simulink model "MCU_FOC"  (R2022b)
settings: Solver=FixedStepDiscrete  StartTime=0.0  StopTime=10.0  FixedStep=0.0001  RelTol=1e-3
values from neighbouring files (symbols this model uses):
  C_FOC_DecoupleEn_u8 = 0.0    [MCU_FOC_Sldd.sldd]    (also in MCU_FOC_Sldd_objects.m = myPackage.Parameter)
  C_FOC_DecoupleUdCoeff_f32 = 0.0    [MCU_FOC_Sldd.sldd]    (also in MCU_FOC_Sldd_objects.m = myPackage.Parameter)
  C_FOC_DecoupleUeCoeff_f32 = 0.0    [MCU_FOC_Sldd.sldd]    (also in MCU_FOC_Sldd_objects.m = myPackage.Parameter)
  C_FOC_DecoupleUqCoeff_f32 = 0.0    [MCU_FOC_Sldd.sldd]    (also in MCU_FOC_Sldd_objects.m = myPackage.Parameter)
  C_FOC_DPWMEN_u8 = 0.0    [MCU_FOC_Sldd.sldd]    (also in MCU_FOC_Sldd_objects.m = myPackage.Parameter)
  C_FOC_IgnoreShunt_u8 = 0.0    [MCU_FOC_Sldd.sldd]    (also in MCU_FOC_Sldd_objects.m = myPackage.Parameter)
  C_FOC_ThetaOffsetCoeff_f32 = 0.0    [MCU_FOC_Sldd.sldd]    (also in MCU_FOC_Sldd_objects.m = myPackage.Parameter)
undefined symbols (not defined in the file or in its folder): ABC_SAMPLE, ANALOG, cAgeingMode, cParaRecogMode, cSingleBoardMode, cVvvfOpenMode, MAIN_CPU_FRE, ParamCfg_BaseSpeed_u16, ParamCfg_CommandSource_u16, ParamCfg_IdKi_u16, ParamCfg_IdKp_u16, ParamCfg_IdStep1_u16, ParamCfg_IdStep2_u16, ParamCfg_IqKi_u16, ParamCfg_IqKp_u16, ParamCfg_IqStep_u16, ParamCfg_MotorLsd_u16, ParamCfg_MotorNp_u16, ParamCfg_MotorUlsq_u16, ParamCfg_PwmFreqHigh_u16, ParamCfg_PwmFreqLow_u16, ParamCfg_Pwmprdchgen_u16, ParamCfg_RotateNp_u16, ParamCfg_RotorFlux_u16, ParamCfg_SampleMode_u16, TESTBED
libraries: simulink x40, YS_UserDefined_Library x17
(part 1 of 2)
settings Model: DataDictionary=MCU_FOC_Sldd.sldd  Creator=ZYH  LastModifiedBy=ZYH
settings OptimizationCC: DefaultParameterBehavior=Inlined  EnhancedBackFolding=on  PassReuseOutputArgsAs=Individual arguments  ZeroExternalMemoryAtStartup=off  ZeroInternalMemoryAtStartup=off  OptimizeBlockOrder=speed  DifferentSizesBufferReuse=on  OptimizationCustomize=off  EfficientTunableParamExpr=on
settings DebuggingCC: ParameterTunabilityLossMsg=error
settings SFSimCC: MATLABDynamicMemAlloc=off
settings RTWCC: Description=Embedded Coder  SystemTargetFile=ert.tlc  GenCodeOnly=on  TemplateMakefile=ert_default_tmf
settings CodeAppCC: ForceParamTrailComments=on  IgnoreCustomStorageClasses=off  OperatorAnnotations=on  SimulinkDataObjDesc=on  SFDataObjDesc=on  InsertBlockDesc=on
settings ERTTargetCC: TargetLangStandard=C99 (ISO)  GenerateSampleERTMain=on  InlinedParameterPlacement=NonHierarchical  ERTCustomFileTemplate=example_file_process.tlc

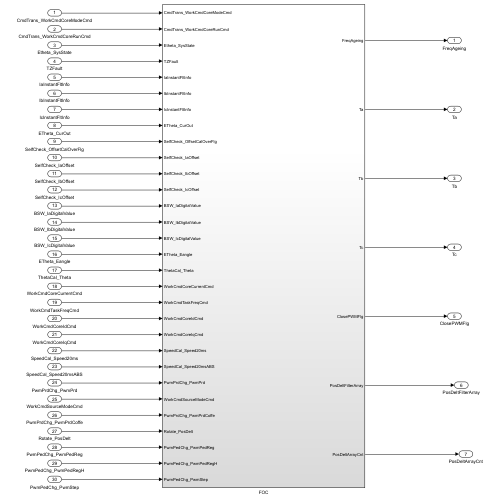
[thumbnail: Simulink's stored preview of the top-level diagram]
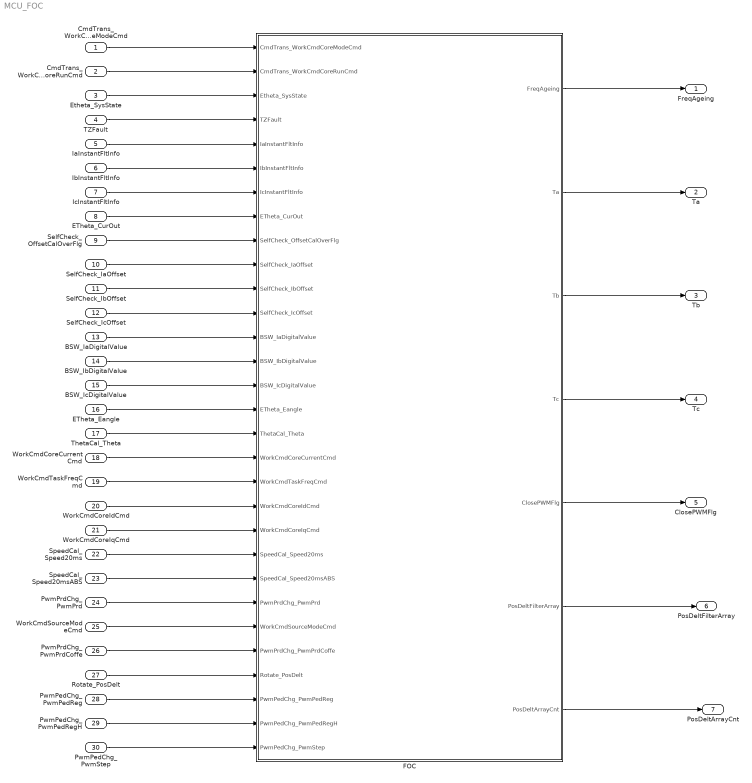
== system MCU_FOC ==
  CmdTrans_WorkCmdCoreModeCmd : Inport
  CmdTrans_WorkCmdCoreRunCmd : Inport  Port=2
  Etheta_SysState : Inport  Port=3
  TZFault : Inport  Port=4
  IaInstantFltInfo : Inport  Port=5
  IbInstantFltInfo : Inport  Port=6
  IcInstantFltInfo : Inport  Port=7
  ETheta_CurOut : Inport  Port=8
  SelfCheck_OffsetCalOverFlg : Inport  Port=9
  SelfCheck_IaOffset : Inport  Port=10
  SelfCheck_IbOffset : Inport  Port=11
  SelfCheck_IcOffset : Inport  Port=12
  BSW_IaDigitalValue : Inport  Port=13
  BSW_IbDigitalValue : Inport  Port=14
  BSW_IcDigitalValue : Inport  Port=15
  ETheta_Eangle : Inport  Port=16
  ThetaCal_Theta : Inport  Port=17
  WorkCmdCoreCurrentCmd : Inport  Port=18
  WorkCmdTaskFreqCmd : Inport  Port=19
  WorkCmdCoreIdCmd : Inport  Port=20
  WorkCmdCoreIqCmd : Inport  Port=21
  SpeedCal_Speed20ms : Inport  Port=22
  SpeedCal_Speed20msABS : Inport  Port=23
  PwmPrdChg_PwmPrd : Inport  Port=24
  WorkCmdSourceModeCmd : Inport  Port=25
  PwmPrdChg_PwmPrdCoffe : Inport  Port=26
  Rotate_PosDelt : Inport  Port=27
  PwmPedChg_PwmPedReg : Inport  Port=28
  PwmPedChg_PwmPedRegH : Inport  Port=29
  PwmPedChg_PwmStep : Inport  Port=30
  FOC : Subsystem
  FreqAgeing : Outport
  Ta : Outport  Port=2
  Tb : Outport  Port=3
  Tc : Outport  Port=4
  ClosePWMFlg : Outport  Port=5
  PosDeltFilterArray : Outport  Port=6
  PosDeltArrayCnt : Outport  Port=7
  wires:
  FOC/2(Ta) -> Ta/1
  WorkCmdCoreIqCmd/1 -> FOC/21(WorkCmdCoreIqCmd)
  WorkCmdCoreCurrentCmd/1 -> FOC/18(WorkCmdCoreCurrentCmd)
  FOC/1(FreqAgeing) -> FreqAgeing/1
  WorkCmdTaskFreqCmd/1 -> FOC/19(WorkCmdTaskFreqCmd)
  SelfCheck_IaOffset/1 -> FOC/10(SelfCheck_IaOffset)
  WorkCmdCoreIdCmd/1 -> FOC/20(WorkCmdCoreIdCmd)
  SelfCheck_IbOffset/1 -> FOC/11(SelfCheck_IbOffset)
  IcInstantFltInfo/1 -> FOC/7(IcInstantFltInfo)
  ETheta_Eangle/1 -> FOC/16(ETheta_Eangle)
  SelfCheck_OffsetCalOverFlg/1 -> FOC/9(SelfCheck_OffsetCalOverFlg)
  ThetaCal_Theta/1 -> FOC/17(ThetaCal_Theta)
  TZFault/1 -> FOC/4(TZFault)
  PwmPedChg_PwmPedReg/1 -> FOC/28(PwmPedChg_PwmPedReg)
  PwmPrdChg_PwmPrd/1 -> FOC/24(PwmPrdChg_PwmPrd)
  Rotate_PosDelt/1 -> FOC/27(Rotate_PosDelt)
  SpeedCal_Speed20ms/1 -> FOC/22(SpeedCal_Speed20ms)
  FOC/4(Tc) -> Tc/1
  BSW_IaDigitalValue/1 -> FOC/13(BSW_IaDigitalValue)
  BSW_IbDigitalValue/1 -> FOC/14(BSW_IbDigitalValue)
  PwmPedChg_PwmPedRegH/1 -> FOC/29(PwmPedChg_PwmPedRegH)
  PwmPrdChg_PwmPrdCoffe/1 -> FOC/26(PwmPrdChg_PwmPrdCoffe)
  WorkCmdSourceModeCmd/1 -> FOC/25(WorkCmdSourceModeCmd)
  ETheta_CurOut/1 -> FOC/8(ETheta_CurOut)
  SpeedCal_Speed20msABS/1 -> FOC/23(SpeedCal_Speed20msABS)
  BSW_IcDigitalValue/1 -> FOC/15(BSW_IcDigitalValue)
  Etheta_SysState/1 -> FOC/3(Etheta_SysState)
  SelfCheck_IcOffset/1 -> FOC/12(SelfCheck_IcOffset)
  IaInstantFltInfo/1 -> FOC/5(IaInstantFltInfo)
  CmdTrans_WorkCmdCoreRunCmd/1 -> FOC/2(CmdTrans_WorkCmdCoreRunCmd)
  IbInstantFltInfo/1 -> FOC/6(IbInstantFltInfo)
  CmdTrans_WorkCmdCoreModeCmd/1 -> FOC/1(CmdTrans_WorkCmdCoreModeCmd)
  FOC/3(Tb) -> Tb/1
  FOC/5(ClosePWMFlg) -> ClosePWMFlg/1
  PwmPedChg_PwmStep/1 -> FOC/30(PwmPedChg_PwmStep)
  FOC/6(PosDeltFilterArray) -> PosDeltFilterArray/1
  FOC/7(PosDeltArrayCnt) -> PosDeltArrayCnt/1

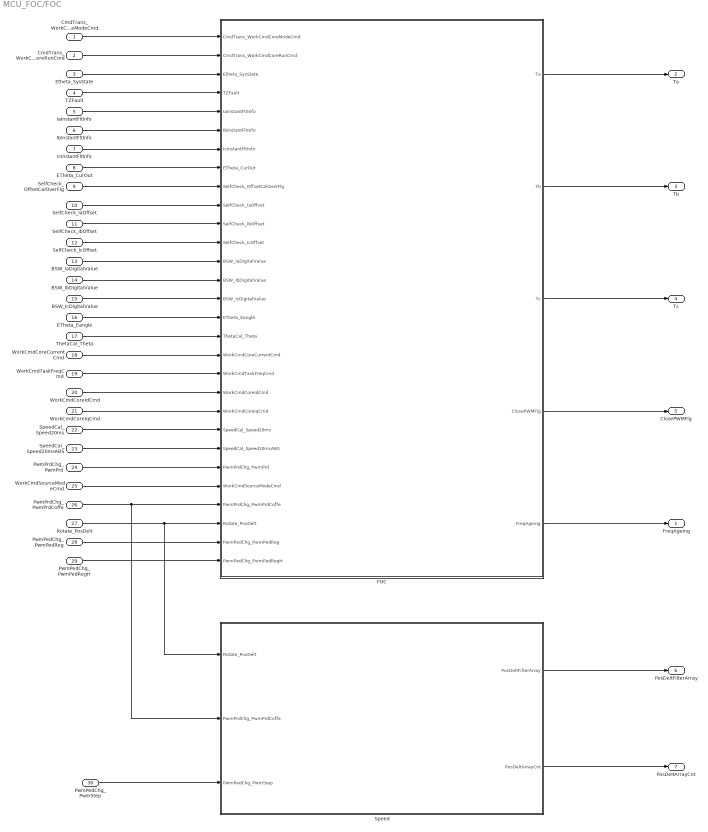
== system MCU_FOC/FOC ==
  CmdTrans_WorkCmdCoreModeCmd : Inport
  CmdTrans_WorkCmdCoreRunCmd : Inport  Port=2
  Etheta_SysState : Inport  Port=3
  TZFault : Inport  Port=4
  IaInstantFltInfo : Inport  Port=5
  IbInstantFltInfo : Inport  Port=6
  IcInstantFltInfo : Inport  Port=7
  ETheta_CurOut : Inport  Port=8
  SelfCheck_OffsetCalOverFlg : Inport  Port=9
  SelfCheck_IaOffset : Inport  Port=10
  SelfCheck_IbOffset : Inport  Port=11
  SelfCheck_IcOffset : Inport  Port=12
  BSW_IaDigitalValue : Inport  Port=13
  BSW_IbDigitalValue : Inport  Port=14
  BSW_IcDigitalValue : Inport  Port=15
  ETheta_Eangle : Inport  Port=16
  ThetaCal_Theta : Inport  Port=17
  WorkCmdCoreCurrentCmd : Inport  Port=18
  WorkCmdTaskFreqCmd : Inport  Port=19
  WorkCmdCoreIdCmd : Inport  Port=20
  WorkCmdCoreIqCmd : Inport  Port=21
  SpeedCal_Speed20ms : Inport  Port=22
  SpeedCal_Speed20msABS : Inport  Port=23
  PwmPrdChg_PwmPrd : Inport  Port=24
  WorkCmdSourceModeCmd : Inport  Port=25
  PwmPrdChg_PwmPrdCoffe : Inport  Port=26
  Rotate_PosDelt : Inport  Port=27
  PwmPedChg_PwmPedReg : Inport  Port=28
  PwmPedChg_PwmPedRegH : Inport  Port=29
  PwmPedChg_PwmStep : Inport  Port=30
  FOC : Subsystem
  Speed : Subsystem
  FreqAgeing : Outport
  Ta : Outport  Port=2
  Tb : Outport  Port=3
  Tc : Outport  Port=4
  ClosePWMFlg : Outport  Port=5
  PosDeltFilterArray : Outport  Port=6
  PosDeltArrayCnt : Outport  Port=7
  wires:
  CmdTrans_WorkCmdCoreModeCmd/1 -> FOC/1(CmdTrans_WorkCmdCoreModeCmd)
  CmdTrans_WorkCmdCoreRunCmd/1 -> FOC/2(CmdTrans_WorkCmdCoreRunCmd)
  Etheta_SysState/1 -> FOC/3(Etheta_SysState)
  TZFault/1 -> FOC/4(TZFault)
  IaInstantFltInfo/1 -> FOC/5(IaInstantFltInfo)
  IbInstantFltInfo/1 -> FOC/6(IbInstantFltInfo)
  IcInstantFltInfo/1 -> FOC/7(IcInstantFltInfo)
  ETheta_CurOut/1 -> FOC/8(ETheta_CurOut)
  SelfCheck_OffsetCalOverFlg/1 -> FOC/9(SelfCheck_OffsetCalOverFlg)
  SelfCheck_IaOffset/1 -> FOC/10(SelfCheck_IaOffset)
  SelfCheck_IbOffset/1 -> FOC/11(SelfCheck_IbOffset)
  SelfCheck_IcOffset/1 -> FOC/12(SelfCheck_IcOffset)
  BSW_IaDigitalValue/1 -> FOC/13(BSW_IaDigitalValue)
  BSW_IbDigitalValue/1 -> FOC/14(BSW_IbDigitalValue)
  BSW_IcDigitalValue/1 -> FOC/15(BSW_IcDigitalValue)
  ETheta_Eangle/1 -> FOC/16(ETheta_Eangle)
  ThetaCal_Theta/1 -> FOC/17(ThetaCal_Theta)
  WorkCmdCoreCurrentCmd/1 -> FOC/18(WorkCmdCoreCurrentCmd)
  WorkCmdTaskFreqCmd/1 -> FOC/19(WorkCmdTaskFreqCmd)
  WorkCmdCoreIdCmd/1 -> FOC/20(WorkCmdCoreIdCmd)
  WorkCmdCoreIqCmd/1 -> FOC/21(WorkCmdCoreIqCmd)
  SpeedCal_Speed20ms/1 -> FOC/22(SpeedCal_Speed20ms)
  SpeedCal_Speed20msABS/1 -> FOC/23(SpeedCal_Speed20msABS)
  PwmPrdChg_PwmPrd/1 -> FOC/24(PwmPrdChg_PwmPrd)
  WorkCmdSourceModeCmd/1 -> FOC/25(WorkCmdSourceModeCmd)
  PwmPrdChg_PwmPrdCoffe/1 -> Speed/2(PwmPrdChg_PwmPrdCoffe), FOC/26(PwmPrdChg_PwmPrdCoffe)
  Rotate_PosDelt/1 -> Speed/1(Rotate_PosDelt), FOC/27(Rotate_PosDelt)
  PwmPedChg_PwmPedReg/1 -> FOC/28(PwmPedChg_PwmPedReg)
  PwmPedChg_PwmPedRegH/1 -> FOC/29(PwmPedChg_PwmPedRegH)
  FOC/1(Ta) -> Ta/1
  FOC/2(Tb) -> Tb/1
  FOC/3(Tc) -> Tc/1
  FOC/4(ClosePWMFlg) -> ClosePWMFlg/1
  FOC/5(FreqAgeing) -> FreqAgeing/1
  PwmPedChg_PwmStep/1 -> Speed/3(PwmPedChg_PwmStep)
  Speed/1(PosDeltFilterArray) -> PosDeltFilterArray/1
  Speed/2(PosDeltArrayCnt) -> PosDeltArrayCnt/1

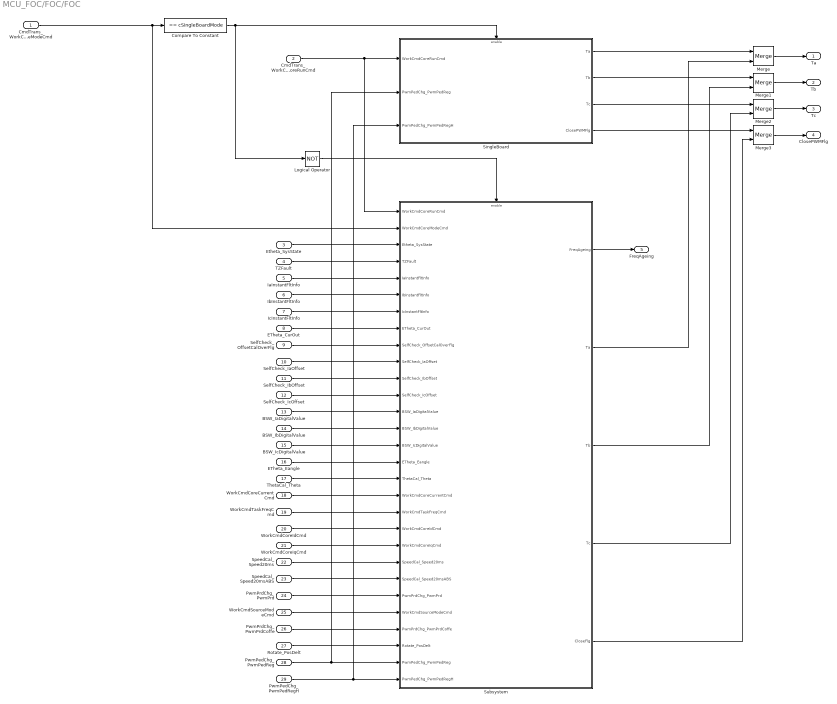
== system MCU_FOC/FOC/FOC ==
  CmdTrans_WorkCmdCoreModeCmd : Inport
  CmdTrans_WorkCmdCoreRunCmd : Inport  Port=2
  Etheta_SysState : Inport  Port=3
  TZFault : Inport  Port=4
  IaInstantFltInfo : Inport  Port=5
  IbInstantFltInfo : Inport  Port=6
  IcInstantFltInfo : Inport  Port=7
  ETheta_CurOut : Inport  Port=8
  SelfCheck_OffsetCalOverFlg : Inport  Port=9
  SelfCheck_IaOffset : Inport  Port=10
  SelfCheck_IbOffset : Inport  Port=11
  SelfCheck_IcOffset : Inport  Port=12
  BSW_IaDigitalValue : Inport  Port=13
  BSW_IbDigitalValue : Inport  Port=14
  BSW_IcDigitalValue : Inport  Port=15
  ETheta_Eangle : Inport  Port=16
  ThetaCal_Theta : Inport  Port=17
  WorkCmdCoreCurrentCmd : Inport  Port=18
  WorkCmdTaskFreqCmd : Inport  Port=19
  WorkCmdCoreIdCmd : Inport  Port=20
  WorkCmdCoreIqCmd : Inport  Port=21
  SpeedCal_Speed20ms : Inport  Port=22
  SpeedCal_Speed20msABS : Inport  Port=23
  PwmPrdChg_PwmPrd : Inport  Port=24
  WorkCmdSourceModeCmd : Inport  Port=25
  PwmPrdChg_PwmPrdCoffe : Inport  Port=26
  Rotate_PosDelt : Inport  Port=27
  PwmPedChg_PwmPedReg : Inport  Port=28
  PwmPedChg_PwmPedRegH : Inport  Port=29
  Compare To Constant : simulink/Logic and Bit Operations/Compare To Constant  relop===  const=cSingleBoardMode  OutDataTypeStr=boolean
  Logical Operator : Logic  Operator=NOT  AllPortsSameDT=off  OutDataTypeStr=boolean
  Merge{,1..3} (4 alike) : Merge
  SingleBoard : Subsystem  TreatAsAtomicUnit=on
  Subsystem : Subsystem
  Ta : Outport
  Tb : Outport  Port=2
  Tc : Outport  Port=3
  ClosePWMFlg : Outport  Port=4
  FreqAgeing : Outport  Port=5
  wires:
  SpeedCal_Speed20ms/1 -> Subsystem/22(SpeedCal_Speed20ms)
  Etheta_SysState/1 -> Subsystem/3(Etheta_SysState)
  WorkCmdCoreIdCmd/1 -> Subsystem/20(WorkCmdCoreIdCmd)
  SelfCheck_OffsetCalOverFlg/1 -> Subsystem/9(SelfCheck_OffsetCalOverFlg)
  SelfCheck_IbOffset/1 -> Subsystem/11(SelfCheck_IbOffset)
  PwmPrdChg_PwmPrdCoffe/1 -> Subsystem/26(PwmPrdChg_PwmPrdCoffe)
  Compare To Constant/1 -> SingleBoard/Enable, Logical Operator/1
  ETheta_Eangle/1 -> Subsystem/16(ETheta_Eangle)
  CmdTrans_WorkCmdCoreModeCmd/1 -> Compare To Constant/1, Subsystem/2(WorkCmdCoreModeCmd)
  SingleBoard/3(Tc) -> Merge2/1
  PwmPedChg_PwmPedRegH/1 -> SingleBoard/3(PwmPedChg_PwmPedRegH), Subsystem/29(PwmPedChg_PwmPedRegH)
  ETheta_CurOut/1 -> Subsystem/8(ETheta_CurOut)
  CmdTrans_WorkCmdCoreRunCmd/1 -> Subsystem/1(WorkCmdCoreRunCmd), SingleBoard/1(WorkCmdCoreRunCmd)
  SelfCheck_IcOffset/1 -> Subsystem/12(SelfCheck_IcOffset)
  WorkCmdTaskFreqCmd/1 -> Subsystem/19(WorkCmdTaskFreqCmd)
  PwmPedChg_PwmPedReg/1 -> SingleBoard/2(PwmPedChg_PwmPedReg), Subsystem/28(PwmPedChg_PwmPedReg)
  SingleBoard/1(Ta) -> Merge/1
  PwmPrdChg_PwmPrd/1 -> Subsystem/24(PwmPrdChg_PwmPrd)
  BSW_IaDigitalValue/1 -> Subsystem/13(BSW_IaDigitalValue)
  BSW_IcDigitalValue/1 -> Subsystem/15(BSW_IcDigitalValue)
  ThetaCal_Theta/1 -> Subsystem/17(ThetaCal_Theta)
  IbInstantFltInfo/1 -> Subsystem/6(IbInstantFltInfo)
  IaInstantFltInfo/1 -> Subsystem/5(IaInstantFltInfo)
  Merge/1 -> Ta/1
  Subsystem/3(Tb) -> Merge1/2
  WorkCmdCoreIqCmd/1 -> Subsystem/21(WorkCmdCoreIqCmd)
  SelfCheck_IaOffset/1 -> Subsystem/10(SelfCheck_IaOffset)
  IcInstantFltInfo/1 -> Subsystem/7(IcInstantFltInfo)
  Logical Operator/1 -> Subsystem/Enable
  WorkCmdCoreCurrentCmd/1 -> Subsystem/18(WorkCmdCoreCurrentCmd)
  Rotate_PosDelt/1 -> Subsystem/27(Rotate_PosDelt)
  TZFault/1 -> Subsystem/4(TZFault)
  SpeedCal_Speed20msABS/1 -> Subsystem/23(SpeedCal_Speed20msABS)
  BSW_IbDigitalValue/1 -> Subsystem/14(BSW_IbDigitalValue)
  Subsystem/4(Tc) -> Merge2/2
  Subsystem/1(FreqAgeing) -> FreqAgeing/1
  SingleBoard/4(ClosePWMFlg) -> Merge3/1
  Subsystem/2(Ta) -> Merge/2
  SingleBoard/2(Tb) -> Merge1/1
  Subsystem/5(CloseFlg) -> Merge3/2
  WorkCmdSourceModeCmd/1 -> Subsystem/25(WorkCmdSourceModeCmd)
  Merge1/1 -> Tb/1
  Merge2/1 -> Tc/1
  Merge3/1 -> ClosePWMFlg/1

== system MCU_FOC/FOC/Speed ==
  Rotate_PosDelt : Inport
  PwmPrdChg_PwmPrdCoffe : Inport  Port=2
  PwmPedChg_PwmStep : Inport  Port=3
  Chart : Stateflow chart  TreatAsAtomicUnit=on
  Data Type Conversion : DataTypeConversion  OutDataTypeStr=uint8  SaturateOnIntegerOverflow=off  RndMeth=Floor
  PosDeltFilterArray : Outport
  PosDeltArrayCnt : Outport  Port=2
  wires:
  PwmPedChg_PwmStep/1 -> Data Type Conversion/1
  Data Type Conversion/1 -> Chart/1(PWMStep)
  PwmPrdChg_PwmPrdCoffe/1 -> Chart/2(PwmPrdchgCoffe)
  Chart/1(PosDeltFilterArray) -> PosDeltFilterArray/1
  Chart/2(PosDeltArrayCnt) -> PosDeltArrayCnt/1
  Rotate_PosDelt/1 -> Chart/3(PosDelt)

== system MCU_FOC/FOC/FOC/SingleBoard ==
  WorkCmdCoreRunCmd : Inport
  PwmPedChg_PwmPedReg : Inport  Port=2
  PwmPedChg_PwmPedRegH : Inport  Port=3
  Enable : EnablePort
  ClosePWM : Subsystem  TreatAsAtomicUnit=on
  Compare To Constant : simulink/Logic and Bit Operations/Compare To Constant  relop===  const=true  OutDataTypeStr=boolean
  Compare To Constant1 : simulink/Logic and Bit Operations/Compare To Constant  relop===  const=false  OutDataTypeStr=boolean
  ForcePWM : Subsystem  TreatAsAtomicUnit=on
  Ta : Outport
  Tb : Outport  Port=2
  Tc : Outport  Port=3
  ClosePWMFlg : Outport  Port=4
  wires:
  WorkCmdCoreRunCmd/1 -> Compare To Constant1/1, Compare To Constant/1
  Compare To Constant/1 -> ForcePWM/Enable
  Compare To Constant1/1 -> ClosePWM/Enable
  PwmPedChg_PwmPedRegH/1 -> ForcePWM/2(PwmPedChg_PwmPedRegH)
  PwmPedChg_PwmPedReg/1 -> ForcePWM/1(PwmPedChg_PwmPedReg)
  ForcePWM/1(Ta) -> Ta/1
  ForcePWM/2(Tb) -> Tb/1
  ForcePWM/3(Tc) -> Tc/1
  ClosePWM/1(ClosePWMFlg) -> ClosePWMFlg/1

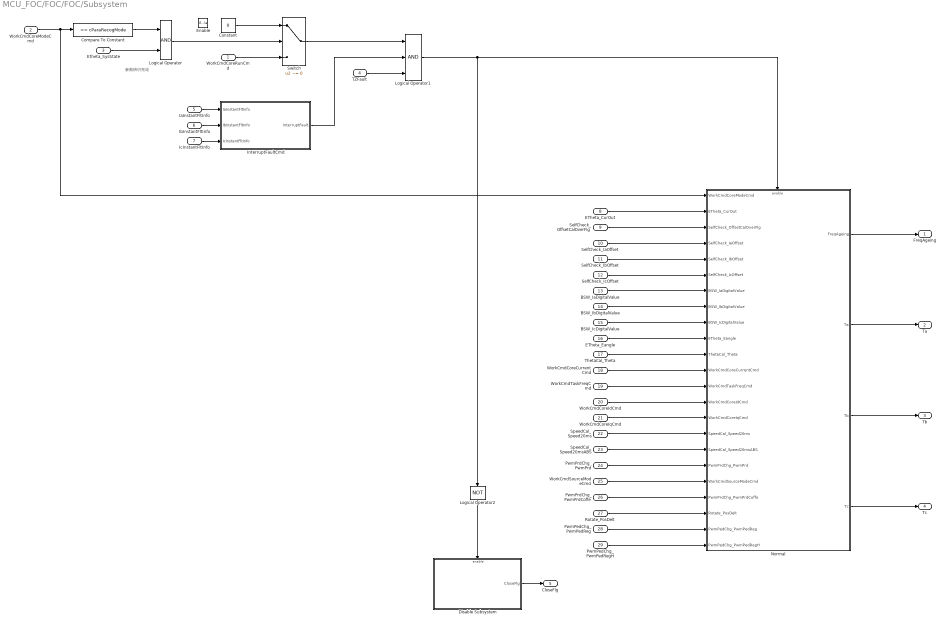
== system MCU_FOC/FOC/FOC/Subsystem ==
  note: 参数辨识完成
  WorkCmdCoreRunCmd : Inport
  WorkCmdCoreModeCmd : Inport  Port=2
  Etheta_SysState : Inport  Port=3
  TZFault : Inport  Port=4
  IaInstantFltInfo : Inport  Port=5
  IbInstantFltInfo : Inport  Port=6
  IcInstantFltInfo : Inport  Port=7
  ETheta_CurOut : Inport  Port=8
  SelfCheck_OffsetCalOverFlg : Inport  Port=9
  SelfCheck_IaOffset : Inport  Port=10
  SelfCheck_IbOffset : Inport  Port=11
  SelfCheck_IcOffset : Inport  Port=12
  BSW_IaDigitalValue : Inport  Port=13
  BSW_IbDigitalValue : Inport  Port=14
  BSW_IcDigitalValue : Inport  Port=15
  ETheta_Eangle : Inport  Port=16
  ThetaCal_Theta : Inport  Port=17
  WorkCmdCoreCurrentCmd : Inport  Port=18
  WorkCmdTaskFreqCmd : Inport  Port=19
  WorkCmdCoreIdCmd : Inport  Port=20
  WorkCmdCoreIqCmd : Inport  Port=21
  SpeedCal_Speed20ms : Inport  Port=22
  SpeedCal_Speed20msABS : Inport  Port=23
  PwmPrdChg_PwmPrd : Inport  Port=24
  WorkCmdSourceModeCmd : Inport  Port=25
  PwmPrdChg_PwmPrdCoffe : Inport  Port=26
  Rotate_PosDelt : Inport  Port=27
  PwmPedChg_PwmPedReg : Inport  Port=28
  PwmPedChg_PwmPedRegH : Inport  Port=29
  Enable : EnablePort
  Compare To Constant : simulink/Logic and Bit Operations/Compare To Constant  relop===  const=cParaRecogMode  OutDataTypeStr=boolean
  Constant : Constant  Value=0  OutDataTypeStr=uint8
  Disable Subsystem : Subsystem  TreatAsAtomicUnit=on
  InterruptFaultCmd : Subsystem
  Logical Operator : Logic  AllPortsSameDT=off  OutDataTypeStr=boolean
  Logical Operator1 : Logic  Inputs=3  AllPortsSameDT=off  OutDataTypeStr=boolean
  Logical Operator2 : Logic  Operator=NOT  Inputs=3  AllPortsSameDT=off  OutDataTypeStr=boolean
  Normal : Subsystem
  Switch : Switch  Criteria=u2 ~= 0  SaturateOnIntegerOverflow=off  InputSameDT=off
  FreqAgeing : Outport
  Ta : Outport  Port=2
  Tb : Outport  Port=3
  Tc : Outport  Port=4
  CloseFlg : Outport  Port=5
  wires:
  Compare To Constant/1 -> Logical Operator/1
  Etheta_SysState/1 -> Logical Operator/2
  Logical Operator/1 -> Switch/2
  Constant/1 -> Switch/1
  WorkCmdCoreRunCmd/1 -> Switch/3
  Switch/1 -> Logical Operator1/1
  InterruptFaultCmd/1(InterruptFault) -> Logical Operator1/2
  TZFault/1 -> Logical Operator1/3
  Logical Operator1/1 -> Logical Operator2/1, Normal/Enable
  Logical Operator2/1 -> Disable Subsystem/Enable
  IaInstantFltInfo/1 -> InterruptFaultCmd/1(IaInstantFltInfo)
  IbInstantFltInfo/1 -> InterruptFaultCmd/2(IbInstantFltInfo)
  IcInstantFltInfo/1 -> InterruptFaultCmd/3(IcInstantFltInfo)
  ETheta_CurOut/1 -> Normal/2(ETheta_CurOut)
  SelfCheck_IbOffset/1 -> Normal/5(SelfCheck_IbOffset)
  SelfCheck_IaOffset/1 -> Normal/4(SelfCheck_IaOffset)
  SelfCheck_IcOffset/1 -> Normal/6(SelfCheck_IcOffset)
  BSW_IaDigitalValue/1 -> Normal/7(BSW_IaDigitalValue)
  SelfCheck_OffsetCalOverFlg/1 -> Normal/3(SelfCheck_OffsetCalOverFlg)
  BSW_IbDigitalValue/1 -> Normal/8(BSW_IbDigitalValue)
  BSW_IcDigitalValue/1 -> Normal/9(BSW_IcDigitalValue)
  WorkCmdCoreModeCmd/1 -> Normal/1(WorkCmdCoreModeCmd), Compare To Constant/1
  ETheta_Eangle/1 -> Normal/10(ETheta_Eangle)
  ThetaCal_Theta/1 -> Normal/11(ThetaCal_Theta)
  WorkCmdCoreCurrentCmd/1 -> Normal/12(WorkCmdCoreCurrentCmd)
  WorkCmdTaskFreqCmd/1 -> Normal/13(WorkCmdTaskFreqCmd)
  WorkCmdCoreIdCmd/1 -> Normal/14(WorkCmdCoreIdCmd)
  WorkCmdCoreIqCmd/1 -> Normal/15(WorkCmdCoreIqCmd)
  WorkCmdSourceModeCmd/1 -> Normal/19(WorkCmdSourceModeCmd)
  PwmPrdChg_PwmPrdCoffe/1 -> Normal/20(PwmPrdChg_PwmPrdCoffe)
  PwmPrdChg_PwmPrd/1 -> Normal/18(PwmPrdChg_PwmPrd)
  SpeedCal_Speed20msABS/1 -> Normal/17(SpeedCal_Speed20msABS)
  SpeedCal_Speed20ms/1 -> Normal/16(SpeedCal_Speed20ms)
  Rotate_PosDelt/1 -> Normal/21(Rotate_PosDelt)
  Normal/1(FreqAgeing) -> FreqAgeing/1
  PwmPedChg_PwmPedReg/1 -> Normal/22(PwmPedChg_PwmPedReg)
  PwmPedChg_PwmPedRegH/1 -> Normal/23(PwmPedChg_PwmPedRegH)
  Normal/2(Ta) -> Ta/1
  Normal/3(Tb) -> Tb/1
  Normal/4(Tc) -> Tc/1
  Disable Subsystem/1(CloseFlg) -> CloseFlg/1

== system MCU_FOC/FOC/FOC/SingleBoard/ClosePWM ==
  Enable : EnablePort
  Constant : Constant  OutDataTypeStr=uint8
  ClosePWMFlg : Outport
  wires:
  Constant/1 -> ClosePWMFlg/1

== system MCU_FOC/FOC/FOC/SingleBoard/ForcePWM ==
  PwmPedChg_PwmPedReg : Inport
  PwmPedChg_PwmPedRegH : Inport  Port=2
  Enable : EnablePort
  CmapA : Constant  Value=1000  OutDataTypeStr=single
  CmapB : Constant  Value=5000  OutDataTypeStr=single
  CmapC : Constant  Value=1000  OutDataTypeStr=single
  Divide : Product  Inputs=*/
  Divide1 : Product  Inputs=*/
  Divide2 : Product  Inputs=*/
  SVPWMCtrl : Subsystem
  Subsystem : Subsystem
  Ta : Outport
  Tb : Outport  Port=2
  Tc : Outport  Port=3
  wires:
  Divide/1 -> SVPWMCtrl/1(CmapA)
  Divide1/1 -> SVPWMCtrl/2(CmapB)
  Divide2/1 -> SVPWMCtrl/3(CmapC)
  CmapB/1 -> Divide1/1
  CmapC/1 -> Divide2/1
  CmapA/1 -> Divide/1
  Subsystem/1(PwmPrdReg) -> Divide2/2, Divide1/2, Divide/2
  PwmPedChg_PwmPedReg/1 -> SVPWMCtrl/4(PwmPedChg_PwmPedReg)
  PwmPedChg_PwmPedRegH/1 -> SVPWMCtrl/5(PwmPedChg_PwmPedRegH)
  SVPWMCtrl/1(Ta) -> Ta/1
  SVPWMCtrl/2(Tb) -> Tb/1
  SVPWMCtrl/3(Tc) -> Tc/1

== system MCU_FOC/FOC/FOC/Subsystem/Disable Subsystem ==
  Enable : EnablePort
  Constant : Constant  OutDataTypeStr=uint8
  CloseFlg : Outport
  wires:
  Constant/1 -> CloseFlg/1

== system MCU_FOC/FOC/FOC/Subsystem/InterruptFaultCmd ==
  IaInstantFltInfo : Inport
  IbInstantFltInfo : Inport  Port=2
  IcInstantFltInfo : Inport  Port=3
  Compare To Zero : simulink/Logic and Bit Operations/Compare To Zero  relop===  OutDataTypeStr=boolean
  Compare To Zero1 : simulink/Logic and Bit Operations/Compare To Zero  relop===  OutDataTypeStr=boolean
  Compare To Zero2 : simulink/Logic and Bit Operations/Compare To Zero  relop===  OutDataTypeStr=boolean
  Logical Operator : Logic  Inputs=3  AllPortsSameDT=off  OutDataTypeStr=boolean
  InterruptFault : Outport
  wires:
  IaInstantFltInfo/1 -> Compare To Zero/1
  IbInstantFltInfo/1 -> Compare To Zero1/1
  IcInstantFltInfo/1 -> Compare To Zero2/1
  Compare To Zero/1 -> Logical Operator/1
  Compare To Zero1/1 -> Logical Operator/2
  Compare To Zero2/1 -> Logical Operator/3
  Logical Operator/1 -> InterruptFault/1

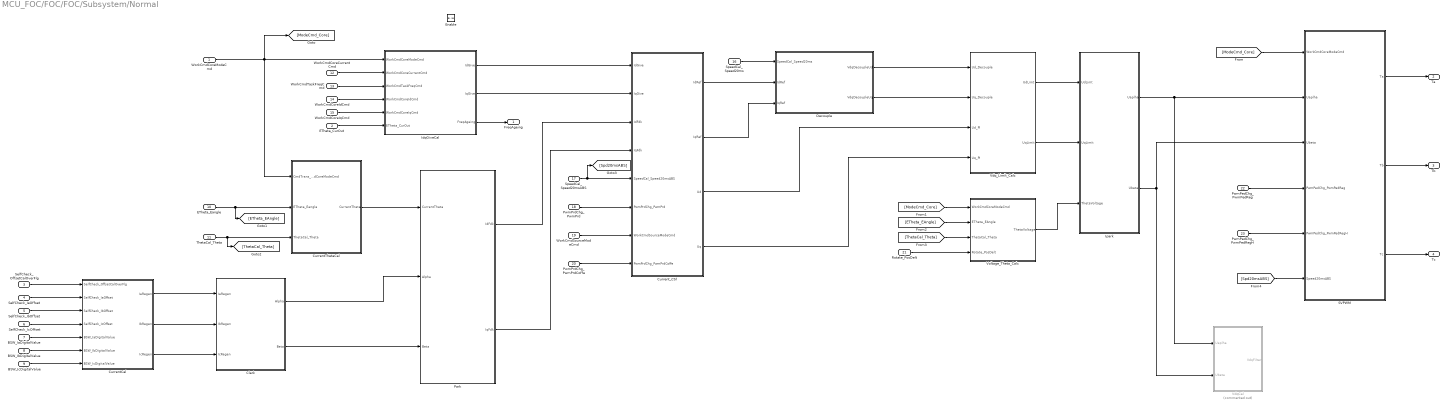
== system MCU_FOC/FOC/FOC/Subsystem/Normal ==
  WorkCmdCoreModeCmd : Inport
  ETheta_CurOut : Inport  Port=2
  SelfCheck_OffsetCalOverFlg : Inport  Port=3
  SelfCheck_IaOffset : Inport  Port=4
  SelfCheck_IbOffset : Inport  Port=5
  SelfCheck_IcOffset : Inport  Port=6
  BSW_IaDigitalValue : Inport  Port=7
  BSW_IbDigitalValue : Inport  Port=8
  BSW_IcDigitalValue : Inport  Port=9
  ETheta_Eangle : Inport  Port=10
  ThetaCal_Theta : Inport  Port=11
  WorkCmdCoreCurrentCmd : Inport  Port=12
  WorkCmdTaskFreqCmd : Inport  Port=13
  WorkCmdCoreIdCmd : Inport  Port=14
  WorkCmdCoreIqCmd : Inport  Port=15
  SpeedCal_Speed20ms : Inport  Port=16
  SpeedCal_Speed20msABS : Inport  Port=17
  PwmPrdChg_PwmPrd : Inport  Port=18
  WorkCmdSourceModeCmd : Inport  Port=19
  PwmPrdChg_PwmPrdCoffe : Inport  Port=20
  Rotate_PosDelt : Inport  Port=21
  PwmPedChg_PwmPedReg : Inport  Port=22
  PwmPedChg_PwmPedRegH : Inport  Port=23
  Enable : EnablePort
  Clark : Subsystem
  CurrentCal : Subsystem
  CurrentThetaCal : Subsystem
  Current_Ctrl : Subsystem
  Decouple : Subsystem
  IdqGiveCal : Subsystem
  Ipark : Subsystem
  Park : Subsystem
  SVPWM : Subsystem
  VdqCal : Subsystem  Commented=on
  Vdq_Limit_Calc : Subsystem
  Voltage_Theta_Calc : Subsystem
  FreqAgeing : Outport
  Ta : Outport  Port=2
  Tb : Outport  Port=3
  Tc : Outport  Port=4
  wires:
  WorkCmdCoreModeCmd/1 -> IdqGiveCal/1(WorkCmdCoreModeCmd), [ModeCmd_Core], CurrentThetaCal/1(CmdTrans_WorkCmdCoreModeCmd)
  IdqGiveCal/1(IdGive) -> Current_Ctrl/1(IdGive)
  Current_Ctrl/3(Ud) -> Vdq_Limit_Calc/3(Ud_PI)
  Current_Ctrl/4(Uq) -> Vdq_Limit_Calc/4(Uq_PI)
  Vdq_Limit_Calc/1(UdLimt) -> Ipark/1(UdLimt)
  Vdq_Limit_Calc/2(UqLimit) -> Ipark/2(UqLimit)
  Voltage_Theta_Calc/1(ThetaVoltage) -> Ipark/3(ThetaVoltage)
  Ipark/1(Uaplha) -> VdqCal/1(Uaplha), SVPWM/2(Uaplha)
  Ipark/2(Ubeta) -> VdqCal/2(Ubeta), SVPWM/3(Ubeta)
  CurrentThetaCal/1(CurrentTheta) -> Park/1(CurrentTheta)
  CurrentCal/1(IaRegen) -> Clark/1(IaRegen)
  CurrentCal/2(IbRegen) -> Clark/2(IbRegen)
  CurrentCal/3(IcRegen) -> Clark/3(IcRegen)
  Clark/2(Beta) -> Park/3(Beta)
  Clark/1(Alpha) -> Park/2(Alpha)
  SelfCheck_OffsetCalOverFlg/1 -> CurrentCal/1(SelfCheck_OffsetCalOverFlg)
  SelfCheck_IbOffset/1 -> CurrentCal/3(SelfCheck_IbOffset)
  SelfCheck_IcOffset/1 -> CurrentCal/4(SelfCheck_IcOffset)
  BSW_IaDigitalValue/1 -> CurrentCal/5(BSW_IaDigitalValue)
  SelfCheck_IaOffset/1 -> CurrentCal/2(SelfCheck_IaOffset)
  BSW_IcDigitalValue/1 -> CurrentCal/7(BSW_IcDigitalValue)
  BSW_IbDigitalValue/1 -> CurrentCal/6(BSW_IbDigitalValue)
  ETheta_Eangle/1 -> CurrentThetaCal/2(ETheta_Eangle), [ETheta_EAngle]
  ThetaCal_Theta/1 -> [ThetaCal_Theta], CurrentThetaCal/3(ThetaCal_Theta)
  ETheta_CurOut/1 -> IdqGiveCal/6(ETheta_CurOut)
  WorkCmdTaskFreqCmd/1 -> IdqGiveCal/3(WorkCmdTaskFreqCmd)
  WorkCmdCoreCurrentCmd/1 -> IdqGiveCal/2(WorkCmdCoreCurrentCmd)
  WorkCmdCoreIdCmd/1 -> IdqGiveCal/4(WorkCmdCoreIdCmd)
  WorkCmdCoreIqCmd/1 -> IdqGiveCal/5(WorkCmdCoreIqCmd)
  IdqGiveCal/2(IqGive) -> Current_Ctrl/2(IqGive)
  IdqGiveCal/3(FreqAgeing) -> FreqAgeing/1
  Park/1(IdFdk) -> Current_Ctrl/3(IdFdk)
  Park/2(IqFdk) -> Current_Ctrl/4(IqFdk)
  SpeedCal_Speed20ms/1 -> Decouple/1(SpeedCal_Speed20ms)
  Current_Ctrl/1(IdRef) -> Decouple/2(IdRef)
  Current_Ctrl/2(IqRef) -> Decouple/3(IqRef)
  PwmPrdChg_PwmPrdCoffe/1 -> Current_Ctrl/8(PwmPrdChg_PwmPrdCoffe)
  SpeedCal_Speed20msABS/1 -> [Spd20msABS], Current_Ctrl/5(SpeedCal_Speed20msABS)
  PwmPrdChg_PwmPrd/1 -> Current_Ctrl/6(PwmPrdChg_PwmPrd)
  WorkCmdSourceModeCmd/1 -> Current_Ctrl/7(WorkCmdSourceModeCmd)
  Decouple/1(VdqDecoupleUd) -> Vdq_Limit_Calc/1(Ud_Decouple)
  Decouple/2(VdqDecoupleUq) -> Vdq_Limit_Calc/2(Uq_Decouple)
  [ModeCmd_Core] -> SVPWM/1(WorkCmdCoreModeCmd)
  [ModeCmd_Core] -> Voltage_Theta_Calc/1(WorkCmdCoreModeCmd)
  [ETheta_EAngle] -> Voltage_Theta_Calc/2(ETheta_EAngle)
  [ThetaCal_Theta] -> Voltage_Theta_Calc/3(ThetaCal_Theta)
  Rotate_PosDelt/1 -> Voltage_Theta_Calc/4(Rotate_PosDelt)
  PwmPedChg_PwmPedReg/1 -> SVPWM/4(PwmPedChg_PwmPedReg)
  PwmPedChg_PwmPedRegH/1 -> SVPWM/5(PwmPedChg_PwmPedRegH)
  SVPWM/1(Ta) -> Ta/1
  SVPWM/2(Tb) -> Tb/1
  SVPWM/3(Tc) -> Tc/1
  [Spd20msABS] -> SVPWM/6(Speed20msABS)

== system MCU_FOC/FOC/FOC/SingleBoard/ForcePWM/SVPWMCtrl ==
  CmapA : Inport
  CmapB : Inport  Port=2
  CmapC : Inport  Port=3
  PwmPedChg_PwmPedReg : Inport  Port=4
  PwmPedChg_PwmPedRegH : Inport  Port=5
  Data Type Conversion : DataTypeConversion  OutDataTypeStr=uint16  SaturateOnIntegerOverflow=off  RndMeth=Floor
  Data Type Conversion1 : DataTypeConversion  OutDataTypeStr=uint16  SaturateOnIntegerOverflow=off  RndMeth=Floor
  Data Type Conversion2 : DataTypeConversion  OutDataTypeStr=uint16  SaturateOnIntegerOverflow=off  RndMeth=Floor
  DynamicSaturation : YS_UserDefined_Library/Saturation/DynamicSaturation
      settings: SourceProductName=YS
  DynamicSaturation1 : YS_UserDefined_Library/Saturation/DynamicSaturation
      settings: SourceProductName=YS
  DynamicSaturation2 : YS_UserDefined_Library/Saturation/DynamicSaturation
      settings: SourceProductName=YS
  PWM_PERIOD_L : Constant  Value=700  OutDataTypeStr=uint16
  Product : Product
  Product1 : Product
  Product2 : Product
  Ta : Outport
  Tb : Outport  Port=2
  Tc : Outport  Port=3
  wires:
  CmapA/1 -> Product/1
  CmapC/1 -> Product2/1
  CmapB/1 -> Product1/1
  PwmPedChg_PwmPedReg/1 -> Product/2, Product1/2, Product2/2
  Product/1 -> Data Type Conversion/1
  Product1/1 -> Data Type Conversion1/1
  Product2/1 -> Data Type Conversion2/1
  Data Type Conversion/1 -> DynamicSaturation/2
  PwmPedChg_PwmPedRegH/1 -> DynamicSaturation2/1, DynamicSaturation1/1, DynamicSaturation/1
  PWM_PERIOD_L/1 -> DynamicSaturation2/3, DynamicSaturation1/3, DynamicSaturation/3
  Data Type Conversion1/1 -> DynamicSaturation1/2
  Data Type Conversion2/1 -> DynamicSaturation2/2
  DynamicSaturation1/1 -> Tb/1
  DynamicSaturation/1 -> Ta/1
  DynamicSaturation2/1 -> Tc/1

== system MCU_FOC/FOC/FOC/SingleBoard/ForcePWM/Subsystem ==
  Constant46 : Constant  Value=ParamCfg_Pwmprdchgen_u16  OutDataTypeStr=uint16
  Constant47 : Constant  Value=ParamCfg_PwmFreqLow_u16  OutDataTypeStr=uint16
  Constant48 : Constant  Value=ParamCfg_PwmFreqHigh_u16  OutDataTypeStr=uint16
  Constant52 : Constant  OutDataTypeStr=single
  Constant53 : Constant  Value=MAIN_CPU_FRE  OutDataTypeStr=uint16
  Constant54 : Constant  Value=1000000  OutDataTypeStr=single
  Divide11 : Product  Inputs=*/
  Gain3 : Gain  Gain=0.5  ParamDataTypeStr=single  OutDataTypeStr=single
  PWM_DEF_LIMIT : Constant  Value=6000  OutDataTypeStr=uint16
  PWM_HIGH_LIMIT : Constant  Value=14000  OutDataTypeStr=uint16
  "PWM_LOW_LIMIT " : Constant  Value=1000  OutDataTypeStr=uint16
  Product17 : Product  Inputs=3  OutDataTypeStr=uint16
  Relational Operator2 : RelationalOperator  Operator=>  OutDataTypeStr=boolean  RndMeth=Simplest  InputSameDT=off
  Relational Operator3 : RelationalOperator  Operator=<  OutDataTypeStr=boolean  RndMeth=Simplest  InputSameDT=off
  Switch11 : Switch  Criteria=u2 ~= 0  SaturateOnIntegerOverflow=off  InputSameDT=off
  Switch12 : Switch  Criteria=u2 ~= 0  SaturateOnIntegerOverflow=off  InputSameDT=off
  Switch13 : Switch  Criteria=u2 > Threshold  SaturateOnIntegerOverflow=off  InputSameDT=off
  PwmPrdReg : Outport
  wires:
  Product17/1 -> PwmPrdReg/1
  Constant52/1 -> Divide11/1
  PWM_DEF_LIMIT/1 -> Switch12/1, Switch13/1
  Constant54/1 -> Product17/1
  Divide11/1 -> Gain3/1
  PWM_HIGH_LIMIT/1 -> Relational Operator2/2
  Constant53/1 -> Product17/2
  Relational Operator2/1 -> Switch12/2
  Constant48/1 -> Switch11/3
  Switch11/1 -> Relational Operator2/1, Relational Operator3/1, Switch13/3
  Switch12/1 -> Divide11/2  "PWM_Freq"
  "PWM_LOW_LIMIT "/1 -> Relational Operator3/2
  Gain3/1 -> Product17/3
  Constant47/1 -> Switch11/1
  Constant46/1 -> Switch11/2
  Relational Operator3/1 -> Switch13/2
  Switch13/1 -> Switch12/3

== system MCU_FOC/FOC/FOC/Subsystem/Normal/Clark ==
  IaRegen : Inport
  IbRegen : Inport  Port=2
  IcRegen : Inport  Port=3
  Clark_AB : Subsystem
  Clark_ABC : Subsystem
  Compare To Constant : simulink/Logic and Bit Operations/Compare To Constant  relop===  const=ABC_SAMPLE  OutDataTypeStr=boolean
  Constant : Constant  Value=ParamCfg_SampleMode_u16
  Logical Operator : Logic  Operator=NOT  AllPortsSameDT=off  OutDataTypeStr=boolean
  Merge : Merge
  Merge1 : Merge
  Alpha : Outport
  Beta : Outport  Port=2
  wires:
  Constant/1 -> Compare To Constant/1
  IaRegen/1 -> Clark_AB/1(IaRegen), Clark_ABC/1(IaRegen)
  IbRegen/1 -> Clark_AB/2(IbRegen), Clark_ABC/2(IbRegen)
  IcRegen/1 -> Clark_AB/3(IcRegen), Clark_ABC/3(IcRegen)
  Clark_ABC/1(Alpha) -> Merge/1
  Clark_AB/2(Beta) -> Merge1/2
  Clark_ABC/2(Beta) -> Merge1/1
  Clark_AB/1(Alpha) -> Merge/2
  Merge/1 -> Alpha/1
  Merge1/1 -> Beta/1
  Compare To Constant/1 -> Logical Operator/1, Clark_ABC/Enable
  Logical Operator/1 -> Clark_AB/Enable

== system MCU_FOC/FOC/FOC/Subsystem/Normal/CurrentCal ==
  SelfCheck_OffsetCalOverFlg : Inport
  SelfCheck_IaOffset : Inport  Port=2
  SelfCheck_IbOffset : Inport  Port=3
  SelfCheck_IcOffset : Inport  Port=4
  BSW_IaDigitalValue : Inport  Port=5
  BSW_IbDigitalValue : Inport  Port=6
  BSW_IcDigitalValue : Inport  Port=7
  Enabled Subsystem : Subsystem  TreatAsAtomicUnit=on
  IaRegen : Outport
  IbRegen : Outport  Port=2
  IcRegen : Outport  Port=3
  wires:
  SelfCheck_OffsetCalOverFlg/1 -> Enabled Subsystem/Enable
  SelfCheck_IaOffset/1 -> Enabled Subsystem/4(SelfCheck_IaOffset)
  BSW_IaDigitalValue/1 -> Enabled Subsystem/1(BSW_IaDigitalValue)
  SelfCheck_IbOffset/1 -> Enabled Subsystem/5(SelfCheck_IbOffset)
  SelfCheck_IcOffset/1 -> Enabled Subsystem/6(SelfCheck_IcOffset)
  BSW_IbDigitalValue/1 -> Enabled Subsystem/2(BSW_IbDigitalValue)
  BSW_IcDigitalValue/1 -> Enabled Subsystem/3(BSW_IcDigitalValue)
  Enabled Subsystem/1(IaRegen) -> IaRegen/1
  Enabled Subsystem/2(IbRegen) -> IbRegen/1
  Enabled Subsystem/3(IcRegen) -> IcRegen/1

== system MCU_FOC/FOC/FOC/Subsystem/Normal/CurrentThetaCal ==
  CmdTrans_WorkCmdCoreModeCmd : Inport
  ETheta_Eangle : Inport  Port=2
  ThetaCal_Theta : Inport  Port=3
  Compare To Constant : simulink/Logic and Bit Operations/Compare To Constant  relop===  const=cParaRecogMode  OutDataTypeStr=boolean
  ParaRecogMode : Subsystem  TreatAsAtomicUnit=on
  Switch : Switch  Criteria=u2 ~= 0  SaturateOnIntegerOverflow=off  InputSameDT=off
  CurrentTheta : Outport
  wires:
  CmdTrans_WorkCmdCoreModeCmd/1 -> Compare To Constant/1
  Compare To Constant/1 -> ParaRecogMode/Enable, Switch/2
  ETheta_Eangle/1 -> ParaRecogMode/1(ETheta_Eangle)
  ParaRecogMode/1(CurrentTheta) -> Switch/1
  Switch/1 -> CurrentTheta/1
  ThetaCal_Theta/1 -> Switch/3

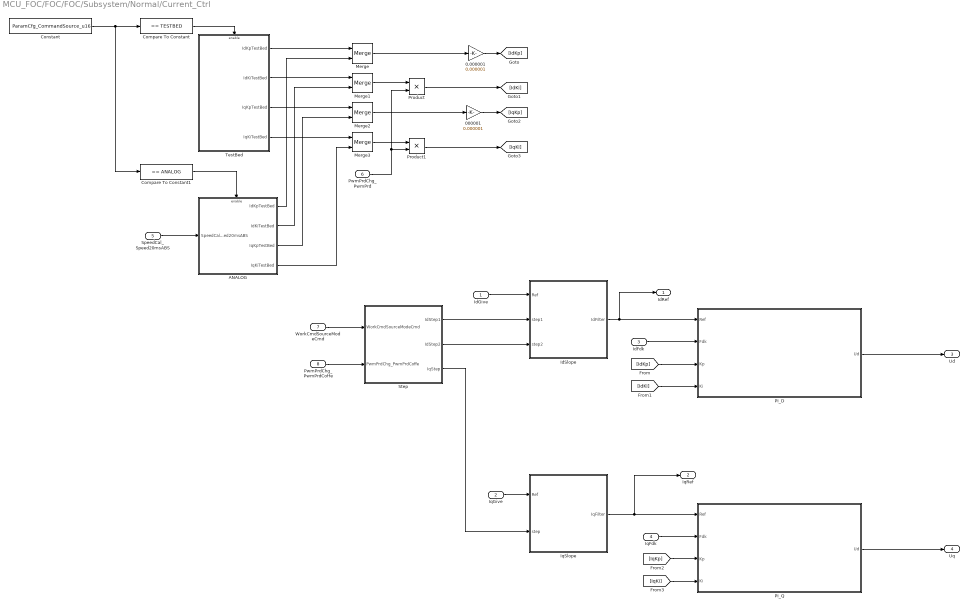
== system MCU_FOC/FOC/FOC/Subsystem/Normal/Current_Ctrl ==
  IdGive : Inport
  IqGive : Inport  Port=2
  IdFdk : Inport  Port=3
  IqFdk : Inport  Port=4
  SpeedCal_Speed20msABS : Inport  Port=5
  PwmPrdChg_PwmPrd : Inport  Port=6
  WorkCmdSourceModeCmd : Inport  Port=7
  PwmPrdChg_PwmPrdCoffe : Inport  Port=8
  0.000001 : Gain  Gain=0.000001  ParamDataTypeStr=single  OutDataTypeStr=single
  000001 : Gain  Gain=0.000001  ParamDataTypeStr=single  OutDataTypeStr=single
  ANALOG : Subsystem  TreatAsAtomicUnit=on
  Compare To Constant : simulink/Logic and Bit Operations/Compare To Constant  relop===  const=TESTBED  OutDataTypeStr=boolean
  Compare To Constant1 : simulink/Logic and Bit Operations/Compare To Constant  relop===  const=ANALOG  OutDataTypeStr=boolean
  Constant : Constant  Value=ParamCfg_CommandSource_u16  OutDataTypeStr=uint16
  IdSlope : Subsystem
  IqSlope : Subsystem
  Merge{,1..3} (4 alike) : Merge
  PI_D : Subsystem
  PI_Q : Subsystem
  Product : Product
  Product1 : Product
  Step : Subsystem
  TestBed : Subsystem  TreatAsAtomicUnit=on
  IdRef : Outport
  IqRef : Outport  Port=2
  Ud : Outport  Port=3
  Uq : Outport  Port=4
  wires:
  Constant/1 -> Compare To Constant1/1, Compare To Constant/1
  Compare To Constant/1 -> TestBed/Enable
  Compare To Constant1/1 -> ANALOG/Enable
  SpeedCal_Speed20msABS/1 -> ANALOG/1(SpeedCal_Speed20msABS)
  TestBed/1(IdKpTestBed) -> Merge/1
  ANALOG/1(IdKpTestBed) -> Merge/2
  TestBed/2(IdKiTestBed) -> Merge1/1
  ANALOG/2(IdKiTestBed) -> Merge1/2
  TestBed/3(IqKpTestBed) -> Merge2/1
  ANALOG/3(IqKpTestBed) -> Merge2/2
  TestBed/4(IqKiTestBed) -> Merge3/1
  ANALOG/4(IqKiTestBed) -> Merge3/2
  Merge/1 -> 0.000001/1
  Merge2/1 -> 000001/1
  Merge1/1 -> Product/1
  PwmPrdChg_PwmPrd/1 -> Product1/2, Product/2
  Merge3/1 -> Product1/1
  PwmPrdChg_PwmPrdCoffe/1 -> Step/2(PwmPrdChg_PwmPrdCoffe)
  WorkCmdSourceModeCmd/1 -> Step/1(WorkCmdSourceModeCmd)
  IdGive/1 -> IdSlope/1(Ref)
  Step/1(IdStep1) -> IdSlope/2(step1)
  Step/2(IdStep2) -> IdSlope/3(step2)
  IqGive/1 -> IqSlope/1(Ref)
  Step/3(IqStep) -> IqSlope/2(step)
  IdFdk/1 -> PI_D/2(Fdk)
  0.000001/1 -> [IdKp]
  000001/1 -> [IqKp]
  Product1/1 -> [IqKi]
  Product/1 -> [IdKi]
  IdSlope/1(IdFilter) -> IdRef/1, PI_D/1(Ref)
  [IdKp] -> PI_D/3(Kp)
  [IdKi] -> PI_D/4(Ki)
  IqFdk/1 -> PI_Q/2(Fdk)
  [IqKp] -> PI_Q/3(Kp)
  [IqKi] -> PI_Q/4(Ki)
  PI_D/1(Ud) -> Ud/1
  PI_Q/1(Ud) -> Uq/1
  IqSlope/1(IqFilter) -> IqRef/1, PI_Q/1(Ref)

== system MCU_FOC/FOC/FOC/Subsystem/Normal/Decouple ==
  note: 端口输出有特殊处理
  SpeedCal_Speed20ms : Inport
  IdRef : Inport  Port=2
  IqRef : Inport  Port=3
  Constant : Constant  Value=C_FOC_DecoupleEn_u8  OutDataTypeStr=uint8
  DecoupleCalc : Subsystem
  VdqDecoupleUd : Outport
  VdqDecoupleUq : Outport  Port=2
  wires:
  SpeedCal_Speed20ms/1 -> DecoupleCalc/1(SpeedCal_Speed20ms)
  IdRef/1 -> DecoupleCalc/2(IdRef)
  IqRef/1 -> DecoupleCalc/3(IqRef)
  DecoupleCalc/1(VdqDecoupleUd) -> VdqDecoupleUd/1
  DecoupleCalc/2(VdqDecoupleUq) -> VdqDecoupleUq/1
  Constant/1 -> DecoupleCalc/Enable

== system MCU_FOC/FOC/FOC/Subsystem/Normal/IdqGiveCal ==
  note: 转速、转矩、电流模式
  WorkCmdCoreModeCmd : Inport
  WorkCmdCoreCurrentCmd : Inport  Port=2
  WorkCmdTaskFreqCmd : Inport  Port=3
  WorkCmdCoreIdCmd : Inport  Port=4
  WorkCmdCoreIqCmd : Inport  Port=5
  ETheta_CurOut : Inport  Port=6
  AgeingMode : Subsystem  TreatAsAtomicUnit=on
  Compare To Constant : simulink/Logic and Bit Operations/Compare To Constant  relop===  const=cParaRecogMode  OutDataTypeStr=boolean
  Compare To Constant1 : simulink/Logic and Bit Operations/Compare To Constant  relop===  const=cAgeingMode  OutDataTypeStr=boolean
  Logical Operator : Logic  Operator=OR  AllPortsSameDT=off  OutDataTypeStr=boolean
  Merge : Merge
  Merge1 : Merge
  ParaRecogMode : Subsystem  TreatAsAtomicUnit=on
  Switch : Switch  Criteria=u2 ~= 0  SaturateOnIntegerOverflow=off  InputSameDT=off
  Switch1 : Switch  Criteria=u2 ~= 0  SaturateOnIntegerOverflow=off  InputSameDT=off
  VvvfMode : Subsystem  Commented=on  TreatAsAtomicUnit=on
  IdGive : Outport
  IqGive : Outport  Port=2
  FreqAgeing : Outport  Port=3
  wires:
  Compare To Constant1/1 -> AgeingMode/Enable, Logical Operator/1
  WorkCmdCoreModeCmd/1 -> Compare To Constant/1, Compare To Constant1/1
  Compare To Constant/1 -> Logical Operator/2, ParaRecogMode/Enable
  WorkCmdCoreCurrentCmd/1 -> AgeingMode/1(WorkCmdCoreCurrentCmd)
  WorkCmdTaskFreqCmd/1 -> AgeingMode/2(WorkCmdTaskFreqCmd)
  WorkCmdCoreIdCmd/1 -> Switch/3, AgeingMode/3(WorkCmdCoreIdCmd)
  WorkCmdCoreIqCmd/1 -> Switch1/3, AgeingMode/4(WorkCmdCoreIqCmd)
  ETheta_CurOut/1 -> ParaRecogMode/1(ETheta_CurOut)
  AgeingMode/1(IdGiveAgeing) -> Merge/1
  Switch/1 -> IdGive/1
  Switch1/1 -> IqGive/1
  AgeingMode/3(FreqAgeing) -> FreqAgeing/1
  ParaRecogMode/1(IdGiveParaRecog) -> Merge/2
  AgeingMode/2(IqAgeing) -> Merge1/1
  ParaRecogMode/2(IqGiveParaRecog) -> Merge1/2
  Logical Operator/1 -> Switch1/2, Switch/2
  Merge/1 -> Switch/1
  Merge1/1 -> Switch1/1

== system MCU_FOC/FOC/FOC/Subsystem/Normal/Ipark ==
  UdLimt : Inport
  UqLimit : Inport  Port=2
  ThetaVoltage : Inport  Port=3
  Cos : Trigonometry  Operator=cos
  Data Type Duplicate : DataTypeDuplicate
  Data Type Duplicate1 : DataTypeDuplicate
  Sin : Trigonometry
  dcos : Product  RndMeth=Simplest  OutDataTypeStr=Inherit: Same as first input
  dsin : Product  RndMeth=Simplest  OutDataTypeStr=Inherit: Same as first input
  qcos : Product  RndMeth=Simplest  OutDataTypeStr=Inherit: Same as first input
  qsin : Product  RndMeth=Simplest  OutDataTypeStr=Inherit: Same as first input
  sum_alpha : Sum  Inputs=|+-  RndMeth=Simplest  OutDataTypeStr=Inherit: Same as first input
  sum_beta : Sum  Inputs=|++  RndMeth=Simplest  OutDataTypeStr=Inherit: Same as first input
  Uaplha : Outport
  Ubeta : Outport  Port=2
  wires:
  Sin/1 -> Data Type Duplicate1/2, qsin/2, dsin/2
  dsin/1 -> sum_beta/2
  Cos/1 -> Data Type Duplicate1/1, dcos/2, qcos/2
  UqLimit/1 -> Data Type Duplicate/2, qcos/1, qsin/1
  sum_alpha/1 -> Uaplha/1
  dcos/1 -> sum_alpha/1
  sum_beta/1 -> Ubeta/1
  qsin/1 -> sum_alpha/2
  qcos/1 -> sum_beta/1
  UdLimt/1 -> Data Type Duplicate/1, dsin/1, dcos/1
  ThetaVoltage/1 -> Sin/1, Cos/1

== system MCU_FOC/FOC/FOC/Subsystem/Normal/Park ==
  CurrentTheta : Inport
  Alpha : Inport  Port=2
  Beta : Inport  Port=3
  Add : Sum
  Minus : Sum  Inputs=-+
  Product{,1..3} (4 alike) : Product
  SinCos : Trigonometry  Operator=sincos  ApproximationMethod=CORDIC
  IdFdk : Outport
  IqFdk : Outport  Port=2
  wires:
  Product2/1 -> Minus/1
  Product3/1 -> Minus/2
  [Alpha] -> Product2/1
  Add/1 -> IdFdk/1
  [Sin] -> Product1/2
  [Cos] -> Product/2
  [Beta] -> Product3/1
  [Sin] -> Product2/2
  Product/1 -> Add/1
  Product1/1 -> Add/2
  [Alpha] -> Product/1
  SinCos/2 -> [Cos]
  Beta/1 -> [Beta]
  [Beta] -> Product1/1
  [Cos] -> Product3/2
  SinCos/1 -> [Sin]
  Minus/1 -> IqFdk/1
  Alpha/1 -> [Alpha]
  CurrentTheta/1 -> SinCos/1

== system MCU_FOC/FOC/FOC/Subsystem/Normal/SVPWM ==
  WorkCmdCoreModeCmd : Inport
  Uaplha : Inport  Port=2
  Ubeta : Inport  Port=3
  PwmPedChg_PwmPedReg : Inport  Port=4
  PwmPedChg_PwmPedRegH : Inport  Port=5
  Speed20msABS : Inport  Port=6
  Compare To Constant : simulink/Logic and Bit Operations/Compare To Constant  relop===  const=cVvvfOpenMode  OutDataTypeStr=boolean
  Enabled Subsystem : Subsystem  TreatAsAtomicUnit=on
  Enabled Subsystem1 : Subsystem  TreatAsAtomicUnit=on
  Logical Operator : Logic  Operator=NOT  AllPortsSameDT=off  OutDataTypeStr=boolean
  Merge : Merge
  Merge1 : Merge
  Subsystem : Subsystem
  Ta : Outport
  Tb : Outport  Port=2
  Tc : Outport  Port=3
  wires:
  WorkCmdCoreModeCmd/1 -> Compare To Constant/1
  Compare To Constant/1 -> Logical Operator/1, Enabled Subsystem/Enable
  Uaplha/1 -> Enabled Subsystem1/1(Uaplha), Enabled Subsystem/1(Uaplha)
  Ubeta/1 -> Enabled Subsystem1/2(Ubeta), Enabled Subsystem/2(Ubeta)
  Logical Operator/1 -> Enabled Subsystem1/Enable
  Enabled Subsystem/1(UalphaVvvvf) -> Merge/1
  Enabled Subsystem1/1(UalphaNormal) -> Merge/2
  Enabled Subsystem1/2(UbetaNormal) -> Merge1/2
  Enabled Subsystem/2(UbetaVvvvf) -> Merge1/1
  Merge/1 -> Subsystem/1(UalphaSVPWM)
  Merge1/1 -> Subsystem/2(UbetaSVPWM)
  PwmPedChg_PwmPedRegH/1 -> Subsystem/4(PwmPedChg_PwmPedRegH)
  PwmPedChg_PwmPedReg/1 -> Subsystem/3(PwmPedChg_PwmPedReg)
  Subsystem/1(Ta) -> Ta/1
  Subsystem/2(Tb) -> Tb/1
  Subsystem/3(Tc) -> Tc/1
  Speed20msABS/1 -> Subsystem/5(Speed20msABS)

== system MCU_FOC/FOC/FOC/Subsystem/Normal/VdqCal ==
  Uaplha : Inport
  Ubeta : Inport  Port=2
  VdqFilter : Outport
  wires:
  Uaplha/1 -> VdqFilter/1

== system MCU_FOC/FOC/FOC/Subsystem/Normal/Vdq_Limit_Calc ==
  Ud_Decouple : Inport
  Uq_Decouple : Inport  Port=2
  Ud_PI : Inport  Port=3
  Uq_PI : Inport  Port=4
  Add : Sum
  Add1 : Sum
  Divide : Product  Inputs=*/
  Power : YS_UserDefined_Library/Math/Power
      settings: SourceProductName=YS
  Product : Product
  Product1 : Product
  Relational Operator : RelationalOperator  Operator=>  OutDataTypeStr=boolean  RndMeth=Simplest  InputSameDT=off
  Switch : Switch  Criteria=u2 ~= 0  SaturateOnIntegerOverflow=off  InputSameDT=off
  UsMax : Constant  OutDataTypeStr=single
  UdLimt : Outport
  UqLimit : Outport  Port=2
  wires:
  Add1/1 -> Power/2, Product1/2
  Add/1 -> Power/1, Product/1
  Uq_PI/1 -> Add/1
  Ud_Decouple/1 -> Add/2
  Uq_Decouple/1 -> Add1/1
  Ud_PI/1 -> Add1/2
  Power/1 -> Divide/2, Relational Operator/1
  UsMax/1 -> Switch/3, Divide/1, Relational Operator/2
  Relational Operator/1 -> Switch/2
  Divide/1 -> Switch/1
  Switch/1 -> Product1/1, Product/2  "LimitCoeff"
  Product/1 -> UqLimit/1
  Product1/1 -> UdLimt/1

== system MCU_FOC/FOC/FOC/Subsystem/Normal/Voltage_Theta_Calc ==
  WorkCmdCoreModeCmd : Inport
  ETheta_EAngle : Inport  Port=2
  ThetaCal_Theta : Inport  Port=3
  Rotate_PosDelt : Inport  Port=4
  Compare To Constant : simulink/Logic and Bit Operations/Compare To Constant  relop===  const=cParaRecogMode  OutDataTypeStr=boolean
  Compare To Constant1 : simulink/Logic and Bit Operations/Compare To Constant  relop===  const=cAgeingMode  OutDataTypeStr=boolean
  Constant : Constant  Value=C_FOC_ThetaOffsetCoeff_f32
  Constant1 : Constant
  Constant2 : Constant  Value=ParamCfg_MotorNp_u16  OutDataTypeStr=uint16
  Constant3 : Constant  Value=ParamCfg_RotateNp_u16  OutDataTypeStr=uint16
  Divide : Product  Inputs=*/
  Divide1 : Product  Inputs=*/
  Mapping : YS_UserDefined_Library/Others/Mapping
      settings: SourceProductName=YS
  Product : Product  Inputs=4
  Shift Arithmetic : ArithShift  BitShiftNumber=12  BitShiftDirection=Left
  Switch : Switch  Criteria=u2 ~= 0  SaturateOnIntegerOverflow=off  InputSameDT=off
  Switch1 : Switch  Criteria=u2 ~= 0  SaturateOnIntegerOverflow=off  InputSameDT=off
  ThetaVoltage : Outport
  wires:
  WorkCmdCoreModeCmd/1 -> Compare To Constant1/1, Compare To Constant/1
  Compare To Constant/1 -> Switch/2
  ETheta_EAngle/1 -> Switch/1
  Switch1/1 -> Switch/3
  Compare To Constant1/1 -> Switch1/2
  ThetaCal_Theta/1 -> Switch1/1
  Switch/1 -> Mapping/1
  Mapping/1 -> ThetaVoltage/1
  Constant1/1 -> Shift Arithmetic/1, Divide/1
  Shift Arithmetic/1 -> Divide/2
  Divide/1 -> Product/3
  Constant2/1 -> Divide1/1
  Constant3/1 -> Divide1/2
  Constant/1 -> Product/1
  Rotate_PosDelt/1 -> Product/2
  Divide1/1 -> Product/4
  Product/1 -> Switch1/3

== system MCU_FOC/FOC/FOC/Subsystem/Normal/Clark/Clark_AB ==
  IaRegen : Inport
  IbRegen : Inport  Port=2
  IcRegen : Inport  Port=3
  Enable : EnablePort
  Data Type Duplicate : DataTypeDuplicate
  Terminator : Terminator
  a_plus_2b : Sum  Inputs=+++  RndMeth=Simplest  OutDataTypeStr=Inherit: Same as first input
  one_by_sqrt3 : Gain  Gain=1/sqrt(3)  RndMeth=Simplest  OutDataTypeStr=Inherit: Same as input
  Alpha : Outport
  Beta : Outport  Port=2
  wires:
  IaRegen/1 -> Data Type Duplicate/1, Alpha/1, a_plus_2b/1
  a_plus_2b/1 -> one_by_sqrt3/1
  IbRegen/1 -> Data Type Duplicate/2, a_plus_2b/3, a_plus_2b/2
  one_by_sqrt3/1 -> Beta/1
  IcRegen/1 -> Terminator/1

== system MCU_FOC/FOC/FOC/Subsystem/Normal/Clark/Clark_ABC ==
  IaRegen : Inport
  IbRegen : Inport  Port=2
  IcRegen : Inport  Port=3
  Enable : EnablePort
  Add : Sum
  Data Type Conversion : DataTypeConversion  OutDataTypeStr=single  SaturateOnIntegerOverflow=off  RndMeth=Floor
  Data Type Conversion1 : DataTypeConversion  OutDataTypeStr=single  SaturateOnIntegerOverflow=off  RndMeth=Floor
  Data Type Conversion2 : DataTypeConversion  OutDataTypeStr=single  SaturateOnIntegerOverflow=off  RndMeth=Floor
  Gain : Gain  Gain=1/3  OutDataTypeStr=single
  Gain1 : Gain  Gain=sqrt(3)/3  OutDataTypeStr=single
  Gain2 : Gain  Gain=sqrt(3)/3  OutDataTypeStr=single
  Minus : Sum  Inputs=+--
  Shift Arithmetic : ArithShift  BitShiftNumber=1  BitShiftDirection=Left
  Alpha : Outport
  Beta : Outport  Port=2
  wires:
  Data Type Conversion1/1 -> Gain2/1, Minus/2
  Gain1/1 -> Add/2
  Data Type Conversion2/1 -> Gain1/1, Minus/3
  Minus/1 -> Gain/1
  Gain2/1 -> Add/1
  Gain/1 -> Alpha/1
  Add/1 -> Beta/1
  Data Type Conversion/1 -> Shift Arithmetic/1
  Shift Arithmetic/1 -> Minus/1
  IaRegen/1 -> Data Type Conversion/1
  IbRegen/1 -> Data Type Conversion1/1
  IcRegen/1 -> Data Type Conversion2/1

== system MCU_FOC/FOC/FOC/Subsystem/Normal/CurrentCal/Enabled Subsystem ==
  BSW_IaDigitalValue : Inport
  BSW_IbDigitalValue : Inport  Port=2
  BSW_IcDigitalValue : Inport  Port=3
  SelfCheck_IaOffset : Inport  Port=4
  SelfCheck_IbOffset : Inport  Port=5
  SelfCheck_IcOffset : Inport  Port=6
  Enable : EnablePort
  Constant : Constant  Value=C_FOC_IgnoreShunt_u8
  CurrentRegen : Subsystem
  Minus : Sum  Inputs=+-
  Minus1 : Sum  Inputs=+-
  Minus2 : Sum  Inputs=+-
  IaRegen : Outport
  IbRegen : Outport  Port=2
  IcRegen : Outport  Port=3
  wires:
  BSW_IaDigitalValue/1 -> Minus/1
  SelfCheck_IaOffset/1 -> Minus/2
  SelfCheck_IbOffset/1 -> Minus1/2
  BSW_IbDigitalValue/1 -> Minus1/1
  BSW_IcDigitalValue/1 -> Minus2/1
  SelfCheck_IcOffset/1 -> Minus2/2
  Minus/1 -> CurrentRegen/2(Ia)
  Minus1/1 -> CurrentRegen/3(Ib)
  Minus2/1 -> CurrentRegen/4(Ic)
  Constant/1 -> CurrentRegen/1(IgnoreShunt)
  CurrentRegen/1(IaRegen) -> IaRegen/1
  CurrentRegen/2(IbRegen) -> IbRegen/1
  CurrentRegen/3(IcRegen) -> IcRegen/1

== system MCU_FOC/FOC/FOC/Subsystem/Normal/CurrentThetaCal/ParaRecogMode ==
  ETheta_Eangle : Inport
  Enable : EnablePort
  Mapping : YS_UserDefined_Library/Others/Mapping
      settings: SourceProductName=YS
  CurrentTheta : Outport
  wires:
  ETheta_Eangle/1 -> Mapping/1
  Mapping/1 -> CurrentTheta/1

== system MCU_FOC/FOC/FOC/Subsystem/Normal/Current_Ctrl/ANALOG ==
  SpeedCal_Speed20msABS : Inport
  Enable : EnablePort
  Compare To Constant : simulink/Logic and Bit Operations/Compare To Constant  relop=<  const=500  OutDataTypeStr=boolean
  Constant : Constant  Value=300  OutDataTypeStr=single
  Constant1 : Constant  Value=500  OutDataTypeStr=single
  Gain : Gain  Gain=2  ParamDataTypeStr=single  OutDataTypeStr=single
  Switch : Switch  Criteria=u2 > Threshold  SaturateOnIntegerOverflow=off  InputSameDT=off
  IdKpTestBed : Outport
  IdKiTestBed : Outport  Port=2
  IqKpTestBed : Outport  Port=3
  IqKiTestBed : Outport  Port=4
  wires:
  Constant/1 -> IqKiTestBed/1, IdKiTestBed/1
  Switch/1 -> IqKpTestBed/1, IdKpTestBed/1
  SpeedCal_Speed20msABS/1 -> Gain/1
  Gain/1 -> Switch/3, Compare To Constant/1
  Compare To Constant/1 -> Switch/2
  Constant1/1 -> Switch/1

== system MCU_FOC/FOC/FOC/Subsystem/Normal/Current_Ctrl/IdSlope ==
  Ref : Inport  PortDimensions=1
  step1 : Inport  Port=2  PortDimensions=1
  step2 : Inport  Port=3  PortDimensions=1
  Add : Sum
  Gain : Gain  Gain=-1  ParamDataTypeStr=single  OutDataTypeStr=single
  Minus : Sum  Inputs=+-
  Minus1 : Sum  Inputs=+-
  Relational Operator : RelationalOperator  Operator=>  OutDataTypeStr=boolean  RndMeth=Simplest  InputSameDT=off
  Relational Operator1 : RelationalOperator  Operator=<  OutDataTypeStr=boolean  RndMeth=Simplest  InputSameDT=off
  Switch : Switch  Criteria=u2 ~= 0  SaturateOnIntegerOverflow=off  InputSameDT=off
  Switch1 : Switch  Criteria=u2 ~= 0  SaturateOnIntegerOverflow=off  InputSameDT=off
  Unit Delay : UnitDelay  SampleTime=-1  HasFrameUpgradeWarning=on
  IdFilter : Outport
  wires:
  Minus1/1 -> Switch1/1
  step1/1 -> Minus1/2, Add/2, Relational Operator/2
  Switch1/1 -> Switch/3
  Relational Operator1/1 -> Switch1/2
  Switch/1 -> Unit Delay/1, IdFilter/1
  Relational Operator/1 -> Switch/2
  Unit Delay/1 -> Add/1, Minus1/1, Minus/2
  Add/1 -> Switch/1
  Ref/1 -> Switch1/3, Minus/1
  Minus/1 -> Relational Operator1/1, Relational Operator/1
  Gain/1 -> Relational Operator1/2
  step2/1 -> Gain/1

== system MCU_FOC/FOC/FOC/Subsystem/Normal/Current_Ctrl/IqSlope ==
  Ref : Inport  PortDimensions=1
  step : Inport  Port=2  PortDimensions=1
  Add : Sum
  Gain : Gain  Gain=-1  ParamDataTypeStr=single  OutDataTypeStr=single
  Minus : Sum  Inputs=+-  OutDataTypeStr=single
  Minus1 : Sum  Inputs=+-
  Relational Operator : RelationalOperator  Operator=>  OutDataTypeStr=boolean  RndMeth=Simplest  InputSameDT=off
  Relational Operator1 : RelationalOperator  Operator=<  OutDataTypeStr=boolean  RndMeth=Simplest  InputSameDT=off
  Switch : Switch  Criteria=u2 ~= 0  SaturateOnIntegerOverflow=off  InputSameDT=off
  Switch1 : Switch  Criteria=u2 ~= 0  SaturateOnIntegerOverflow=off  InputSameDT=off
  Unit Delay : UnitDelay  SampleTime=-1  HasFrameUpgradeWarning=on
  IqFilter : Outport
  wires:
  Minus1/1 -> Switch1/1
  Switch1/1 -> Switch/3
  Relational Operator1/1 -> Switch1/2
  Switch/1 -> Unit Delay/1, IqFilter/1
  Relational Operator/1 -> Switch/2
  Unit Delay/1 -> Add/1, Minus1/1, Minus/2
  Add/1 -> Switch/1
  Ref/1 -> Switch1/3, Minus/1
  Minus/1 -> Relational Operator1/1, Relational Operator/1
  Gain/1 -> Relational Operator1/2
  step/1 -> Gain/1, Minus1/2, Add/2, Relational Operator/2
